simulink model "num2"  (Simulink 7.4)
settings: Solver=ode45  StartTime=0.0  StopTime=10.0  RelTol=1e-3
settings Model: Creator=autologin  LastModifiedBy=autologin

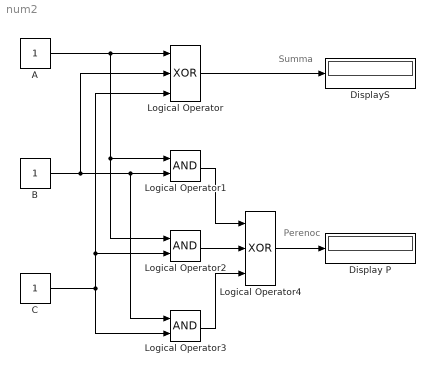
== system num2 ==
  note: Summa
  note: Perenoc
  A : Constant  OutDataType=fixdt(1, 16)  OutScaling=2^0
  B : Constant  OutDataType=fixdt(1, 16)  OutScaling=2^0
  C : Constant  OutDataType=fixdt(1, 16)  OutScaling=2^0
  Display P : Display
  DisplayS : Display
  Logical Operator : Logic  Operator=XOR  Inputs=3  AllPortsSameDT=off  OutDataTypeMode=boolean  LogicDataType=fixdt(0, 8)  OutDataTypeStr=boolean
  Logical Operator1 : Logic  AllPortsSameDT=off  OutDataTypeMode=boolean  LogicDataType=fixdt(0, 8)  OutDataTypeStr=boolean
  Logical Operator2 : Logic  AllPortsSameDT=off  OutDataTypeMode=boolean  LogicDataType=fixdt(0, 8)  OutDataTypeStr=boolean
  Logical Operator3 : Logic  AllPortsSameDT=off  OutDataTypeMode=boolean  LogicDataType=fixdt(0, 8)  OutDataTypeStr=boolean
  Logical Operator4 : Logic  Operator=XOR  Inputs=3  AllPortsSameDT=off  OutDataTypeMode=boolean  LogicDataType=fixdt(0, 8)  OutDataTypeStr=boolean
  wires:
  A/1 -> Logical Operator/1, Logical Operator1/1, Logical Operator2/1
  B/1 -> Logical Operator/2, Logical Operator1/2, Logical Operator3/1
  C/1 -> Logical Operator/3, Logical Operator2/2, Logical Operator3/2
  Logical Operator/1 -> DisplayS/1
  Logical Operator1/1 -> Logical Operator4/1
  Logical Operator2/1 -> Logical Operator4/2
  Logical Operator3/1 -> Logical Operator4/3
  Logical Operator4/1 -> Display P/1
